simulink subsystem "WheelAngVel"  (R2024b)
settings: Solver=VariableStepAuto  StartTime=0.0  StopTime=10.0  RelTol=1e-3
undefined symbols (not defined in the file or in its folder): L, R
settings Model: Creator=Asus  LastModifiedBy=Asus

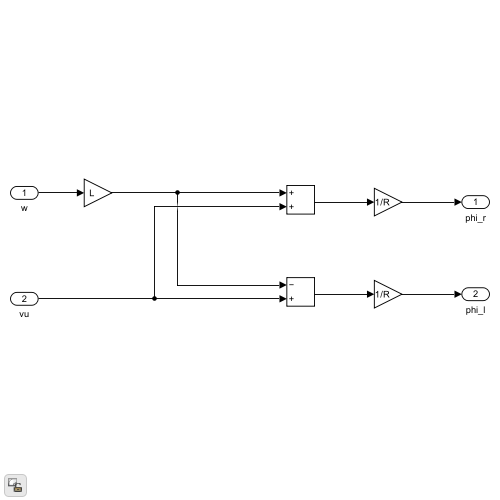
[thumbnail: Simulink's stored preview of the top-level diagram]
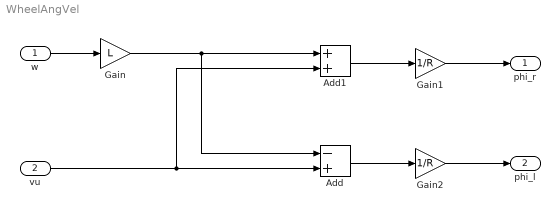
== system WheelAngVel ==
  w : Inport
  vu : Inport  Port=2
  Add : Sum  Inputs=-+
  Add1 : Sum
  Gain : Gain  Gain=L
  Gain1 : Gain  Gain=1/R
  Gain2 : Gain  Gain=1/R
  phi_r : Outport
  phi_l : Outport  Port=2
  wires:
  w/1 -> Gain/1
  Gain/1 -> Add/1, Add1/1
  vu/1 -> Add1/2, Add/2
  Add1/1 -> Gain1/1
  Add/1 -> Gain2/1
  Gain2/1 -> phi_l/1
  Gain1/1 -> phi_r/1
